simulink model "ConSys_A1"  (Simulink 8.3)
settings: Solver=ode3  StartTime=0.0  StopTime=Time(end)  FixedStep=Ts  RelTol=1e-3
values from neighbouring files (symbols this model uses):
  d = r*h    (= 1.6)    [StartUp_A1.m]
  d0 = d*h    (= 0.0032)    [StartUp_A1.m]
  h = 0.002    [StartUp_A1.m]
  Ka = diag([ 3  20  20  150  355  520])    [StartUp_A1.m]
  Kd = diag([ 3   5  25  100   15 1050])    [StartUp_A1.m]
  Ki = diag([35 555 810 7410 1850 5815])    [StartUp_A1.m]
  Kp = diag([55 180 350 1960  680 4450])    [StartUp_A1.m]
  r = 800    [StartUp_A1.m]
  TD = ss(Atd,Btd,Ctd,Dtd,Ts)    [StartUp_A1.m]
  Ts = 1/200    (= 0.005)    [StartUp_A1.m]
undefined symbols (not defined in the file or in its folder): DiscIntNeverNeededParam
undefined symbols (not defined in the file): ADAMS_cwd, ADAMS_exec, ADAMS_host, ADAMS_init, ADAMS_inputs, ADAMS_outputs, ADAMS_prefix, ADAMS_static, ADAMS_sysdir
libraries: cstblocks x6
(part 1 of 9)
settings Model: Creator=baqumau  LastModifiedBy=baqumau
settings SolverCC: SolverResetMethod=Robust  AutoInsertRateTranBlk=on
settings DataIOCC: SignalLoggingSaveFormat=Dataset
settings DebuggingCC: UnderspecifiedInitializationDetection=Simplified  StateNameClashWarn=none
settings GRTTargetCC: CombineOutputUpdateFcns=on  GRTInterface=off

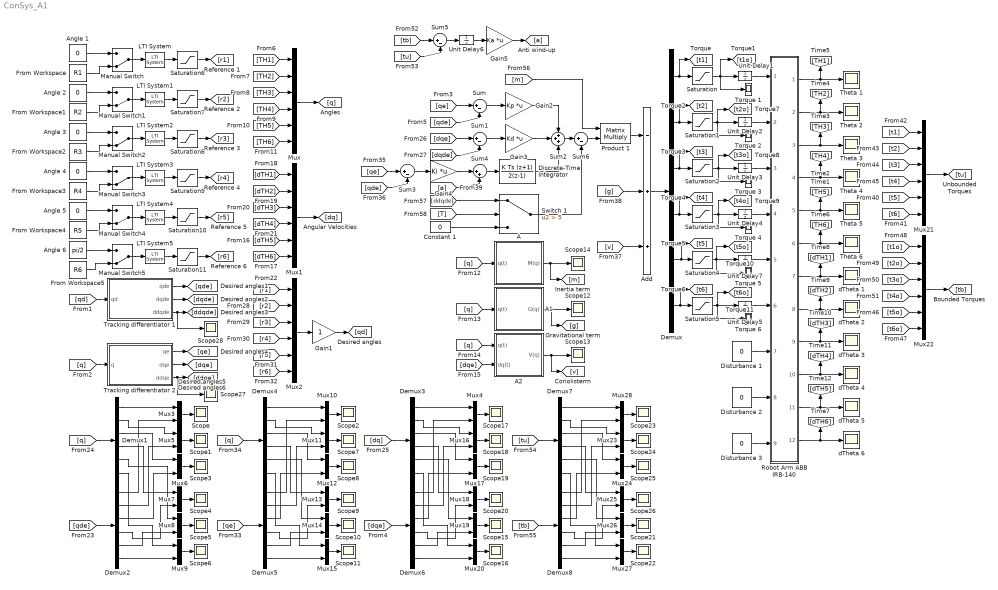
== system ConSys_A1 ==
  A : Subsystem
  A1 : Subsystem
  A2 : Subsystem
  Add : Sum  Inputs=-++
  Angle {1..5} (5 alike) : Constant  Value=0
  Angle 6 : Constant  Value=pi/2
  Constant 1 : Constant  Value=0
  Demux{,1..8} (9 alike) : Demux  Outputs=6
  Discrete-Time Integrator : DiscreteIntegrator  IntegratorMethod=Integration: Trapezoidal  InitialCondition=[0 0 0 0 0 0]'  SampleTime=Ts  ICPrevOutput=DiscIntNeverNeededParam  ICPrevScaledInput=DiscIntNeverNeededParam
  Disturbance 1 : Constant  Value=0
  Disturbance 2 : Constant  Value=0
  Disturbance 3 : Constant  Value=0
  From Workspace : FromWorkspace  VariableName=R1
  From Workspace1 : FromWorkspace  VariableName=R2
  From Workspace2 : FromWorkspace  VariableName=R3
  From Workspace3 : FromWorkspace  VariableName=R4
  From Workspace4 : FromWorkspace  VariableName=R5
  From Workspace5 : FromWorkspace  VariableName=R6
  Gain1 : Gain
  Gain2 : Gain  Gain=Kp  Multiplication=Matrix(K*u)
  Gain3 : Gain  Gain=Kd  Multiplication=Matrix(K*u)
  Gain4 : Gain  Gain=Ki  Multiplication=Matrix(K*u)
  Gain5 : Gain  Gain=Ka  Multiplication=Matrix(K*u)
  LTI System : cstblocks/LTI System  sys=F1z  IC=[]
  LTI System1 : cstblocks/LTI System  sys=F2z  IC=[]
  LTI System2 : cstblocks/LTI System  sys=F3z  IC=[]
  LTI System3 : cstblocks/LTI System  sys=F4z  IC=[]
  LTI System4 : cstblocks/LTI System  sys=F5z  IC=[]
  LTI System5 : cstblocks/LTI System  sys=F6z  IC=[]
  Manual Switch{,1..5} (6 alike) : ManualSwitch  CurrentSetting=0
  Mux{,1..2,21..22} (5 alike) : Mux  Inputs=6
  Mux{3..20,23..28} (24 alike) : Mux  Inputs=2
  Product 1 : Product  Multiplication=Matrix(*)
  Robot Arm ABB IRB-140 : Subsystem
  Saturation : Saturate  UpperLimit=400  LowerLimit=-400
  Saturation1 : Saturate  UpperLimit=300  LowerLimit=-300
  Saturation10 : Saturate  UpperLimit=120  LowerLimit=-120
  Saturation11 : Saturate  UpperLimit=400  LowerLimit=-400
  Saturation2 : Saturate  UpperLimit=250  LowerLimit=-250
  Saturation3 : Saturate  UpperLimit=50  LowerLimit=-50
  Saturation4 : Saturate  UpperLimit=8  LowerLimit=-8
  Saturation5 : Saturate  UpperLimit=0.3  LowerLimit=-0.3
  Saturation6 : Saturate  UpperLimit=180  LowerLimit=-180
  Saturation7 : Saturate  UpperLimit=100  LowerLimit=-100
  Saturation8 : Saturate  UpperLimit=140  LowerLimit=-140
  Saturation9 : Saturate  UpperLimit=200*pi/180  LowerLimit=-200*pi/180
  Scope{,1..28} (29 alike) : Scope
      Scope settings: YMin=-2  YMax=2  SaveName=ScopeData18
      Scope1 settings: YMin=-3  YMax=3  SaveName=ScopeData19
      Scope10 settings: YMin=-2  YMax=2  SaveName=ScopeData20
      Scope11 settings: YMin=-2  SaveName=ScopeData25
      Scope12 settings: YMin=-2  YMax=4  SaveName=ScopeData30
      Scope13 settings: YMin=-2  YMax=4  SaveName=ScopeData31
      Scope14 settings: YMin=-2  YMax=4  SaveName=ScopeData32
      Scope15 settings: YMin=-2  YMax=2  SaveName=ScopeData33
      Scope16 settings: YMin=-2  SaveName=ScopeData34
      Scope17 settings: YMin=-1  YMax=2  SaveName=ScopeData35
      Scope18 settings: YMin=-1  YMax=2  SaveName=ScopeData36
      Scope19 settings: YMin=-1  YMax=2  SaveName=ScopeData37
      Scope2 settings: YMin=-1  YMax=2  SaveName=ScopeData26
      Scope20 settings: YMin=-1  YMax=2  SaveName=ScopeData38
      Scope21 settings: YMin=-2  YMax=2  SaveName=ScopeData39
      Scope22 settings: YMin=-1  YMax=1  SaveName=ScopeData40
      Scope23 settings: YMin=-1  YMax=2  SaveName=ScopeData41
      Scope24 settings: YMin=-1  YMax=2  SaveName=ScopeData42
      Scope25 settings: YMin=-1  YMax=2  SaveName=ScopeData43
      Scope26 settings: YMin=-1  YMax=2  SaveName=ScopeData44
      Scope27 settings: YMin=-2  YMax=2  SaveName=ScopeData45
      Scope28 settings: YMin=-20  YMax=20  SaveName=ScopeData46
      Scope3 settings: YMin=-2  YMax=2  SaveName=ScopeData21
      Scope4 settings: YMin=-2  YMax=2  SaveName=ScopeData22
      Scope5 settings: YMin=-2  YMax=2  SaveName=ScopeData23
      Scope6 settings: SaveName=ScopeData24
      Scope7 settings: YMin=-1  YMax=2  SaveName=ScopeData27
      Scope8 settings: YMin=-1  YMax=2  SaveName=ScopeData28
      Scope9 settings: YMin=-1  YMax=2  SaveName=ScopeData29
  Sum{,1,3,5..6} (5 alike) : Sum  Inputs=|+-
  Sum2 : Sum  Inputs=+++
  Sum4 : Sum  Inputs=|++
  Switch 1 : Switch  Criteria=u2 > Threshold  Threshold=5
  Theta {1..6} (6 alike) : Scope
      Theta 1 settings: YMin=-0.6  YMax=0.6
      Theta 2 settings: YMin=-1  YMax=1  SaveName=ScopeData2
      Theta 3 settings: SaveName=ScopeData3
      Theta 4 settings: SaveName=ScopeData4
      Theta 5 settings: SaveName=ScopeData5
      Theta 6 settings: YMin=-100  YMax=100
  Torque {1..6} (6 alike) : Scope
      Torque 1 settings: YMin=-400  YMax=400  SaveName=ScopeData6
      Torque 2 settings: YMin=-400  YMax=400  SaveName=ScopeData7
      Torque 3 settings: YMin=-400  YMax=400  SaveName=ScopeData8
      Torque 4 settings: YMin=-20  YMax=20  SaveName=ScopeData9
      Torque 5 settings: YMin=-400  YMax=400  SaveName=ScopeData10
      Torque 6 settings: YMin=-0.3  YMax=0.3  SaveName=ScopeData11
  Tracking differentiator 1 : Subsystem
  Tracking differentiator 2 : Subsystem
  Unit Delay{1..7} (7 alike) : UnitDelay  SampleTime=-1
  dTheta {1..6} (6 alike) : Scope
      dTheta 1 settings: SaveName=ScopeData13
      dTheta 2 settings: SaveName=ScopeData14
      dTheta 3 settings: SaveName=ScopeData15
      dTheta 4 settings: SaveName=ScopeData16
      dTheta 5 settings: SaveName=ScopeData17
      dTheta 6 settings: SaveName=ScopeData12
  wires:
  Disturbance 2/1 -> Robot Arm ABB IRB-140/8(Disturbance_2)
  Saturation1/1 -> Torque 2/1, Unit Delay2/1, [t2o]
  Saturation2/1 -> Torque 3/1, Unit Delay3/1, [t3o]
  Saturation3/1 -> Unit Delay4/1, Torque 4/1, [t4o]
  Saturation4/1 -> Unit Delay7/1, [t5o], Torque 5/1
  Saturation5/1 -> Unit Delay5/1, Torque 6/1, [t6o]
  [TH3] -> Mux/3
  [TH6] -> Mux/6
  [TH1] -> Mux/1
  [TH4] -> Mux/4
  [TH5] -> Mux/5
  [TH2] -> Mux/2
  Mux/1 -> [q]
  [q] -> A/1(q(t))
  [q] -> A1/1(q(t))
  [dTH3] -> Mux1/3
  [dTH6] -> Mux1/6
  [dTH1] -> Mux1/1
  [dTH4] -> Mux1/4
  [dTH5] -> Mux1/5
  [dTH2] -> Mux1/2
  Mux1/1 -> [dq]
  Mux2/1 -> Gain1/1
  Demux/1 -> Saturation/1, [t1]
  Demux/2 -> Saturation1/1, [t2]
  Demux/3 -> Saturation2/1, [t3]
  Demux/4 -> Saturation3/1, [t4]
  Demux/6 -> [t6], Saturation5/1
  [qd] -> Tracking differentiator 1/1(qd)
  Tracking differentiator 1/1(qde) -> [qde]
  Tracking differentiator 1/2(dqde) -> [dqde]
  Tracking differentiator 1/3(ddqde) -> Scope28/1, [ddqde]
  [q] -> Demux1/1
  [qde] -> Demux2/1
  Mux3/1 -> Scope/1
  Saturation/1 -> Unit Delay1/1, Torque 1/1, [t1o]
  [q] -> A2/1(q(t))
  [dqe] -> A2/2(dq(t))
  Mux5/1 -> Scope1/1
  Mux6/1 -> Scope3/1
  Mux7/1 -> Scope4/1
  Mux8/1 -> Scope5/1
  Mux9/1 -> Scope6/1
  Demux1/1 -> Mux3/1
  Demux2/1 -> Mux3/2
  Demux1/2 -> Mux5/1
  Demux2/2 -> Mux5/2
  Demux1/3 -> Mux6/1
  Demux2/3 -> Mux6/2
  Demux1/4 -> Mux7/1
  Demux2/4 -> Mux7/2
  Demux1/5 -> Mux8/1
  Demux2/5 -> Mux8/2
  Demux1/6 -> Mux9/1
  Demux2/6 -> Mux9/2
  [r1] -> Mux2/1
  [qe] -> Sum/1
  [qde] -> Sum/2
  Angle 1/1 -> Manual Switch/1
  From Workspace/1 -> Manual Switch/2
  Manual Switch/1 -> LTI System/1
  Angle 2/1 -> Manual Switch1/1
  From Workspace1/1 -> Manual Switch1/2
  Manual Switch1/1 -> LTI System1/1
  Angle 3/1 -> Manual Switch2/1
  From Workspace2/1 -> Manual Switch2/2
  Manual Switch2/1 -> LTI System2/1
  Angle 4/1 -> Manual Switch3/1
  From Workspace3/1 -> Manual Switch3/2
  Manual Switch3/1 -> LTI System3/1
  Angle 5/1 -> Manual Switch4/1
  From Workspace4/1 -> Manual Switch4/2
  Manual Switch4/1 -> LTI System4/1
  Angle 6/1 -> Manual Switch5/1
  From Workspace5/1 -> Manual Switch5/2
  Manual Switch5/1 -> LTI System5/1
  [q] -> Demux4/1
  [qe] -> Demux5/1
  Mux10/1 -> Scope2/1
  Mux11/1 -> Scope7/1
  Mux12/1 -> Scope8/1
  Mux13/1 -> Scope9/1
  Mux14/1 -> Scope10/1
  Mux15/1 -> Scope11/1
  Demux4/1 -> Mux10/1
  Demux5/1 -> Mux10/2
  Demux4/2 -> Mux11/1
  Demux5/2 -> Mux11/2
  Demux4/3 -> Mux12/1
  Demux5/3 -> Mux12/2
  Demux4/4 -> Mux13/1
  Demux5/4 -> Mux13/2
  Demux4/5 -> Mux14/1
  Demux5/5 -> Mux14/2
  Demux4/6 -> Mux15/1
  Demux5/6 -> Mux15/2
  Saturation6/1 -> [r1]
  LTI System/1 -> Saturation6/1
  LTI System1/1 -> Saturation7/1
  LTI System2/1 -> Saturation8/1
  LTI System3/1 -> Saturation9/1
  LTI System4/1 -> Saturation10/1
  LTI System5/1 -> Saturation11/1
  Saturation7/1 -> [r2]
  Saturation8/1 -> [r3]
  Saturation9/1 -> [r4]
  Saturation10/1 -> [r5]
  Saturation11/1 -> [r6]
  Disturbance 1/1 -> Robot Arm ABB IRB-140/7(Disturbance_1)
  Disturbance 3/1 -> Robot Arm ABB IRB-140/9(Disturbance_3)
  [q] -> Tracking differentiator 2/1(q)
  Tracking differentiator 2/1(qe) -> [qe]
  Tracking differentiator 2/2(dqe) -> [dqe]
  Tracking differentiator 2/3(ddqe) -> Scope27/1, [ddqe]
  A1/1(G(q)) -> [g], Scope12/1
  A2/1(V(q)) -> [v], Scope13/1
  A/1(M(q)) -> [m], Scope14/1
  Gain1/1 -> [qd]
  [r2] -> Mux2/2
  [r3] -> Mux2/3
  [r4] -> Mux2/4
  [r5] -> Mux2/5
  [r6] -> Mux2/6
  [dq] -> Demux3/1
  [dqe] -> Demux6/1
  Mux4/1 -> Scope17/1
  Mux16/1 -> Scope18/1
  Mux17/1 -> Scope19/1
  Mux18/1 -> Scope20/1
  Mux19/1 -> Scope15/1
  Mux20/1 -> Scope16/1
  Demux3/1 -> Mux4/1
  Demux6/1 -> Mux4/2
  Demux3/2 -> Mux16/1
  Demux6/2 -> Mux16/2
  Demux3/3 -> Mux17/1
  Demux6/3 -> Mux17/2
  Demux3/4 -> Mux18/1
  Demux6/4 -> Mux18/2
  Demux3/5 -> Mux19/1
  Demux6/5 -> Mux19/2
  Demux3/6 -> Mux20/1
  Demux6/6 -> Mux20/2
  Sum/1 -> Gain2/1
  [dqe] -> Sum1/1
  [dqde] -> Sum1/2
  Sum1/1 -> Gain3/1
  [qe] -> Sum3/1
  [qde] -> Sum3/2
  Unit Delay1/1 -> Robot Arm ABB IRB-140/1(Torque_1)
  Unit Delay2/1 -> Robot Arm ABB IRB-140/2(Torque_2)
  Demux/5 -> [t5], Saturation4/1
  Sum3/1 -> Gain4/1
  Gain4/1 -> Sum4/1
  Sum4/1 -> Discrete-Time Integrator/1
  [a] -> Sum4/2
  [t3] -> Mux21/3
  [t1] -> Mux21/1
  [t4] -> Mux21/4
  [t5] -> Mux21/5
  [t2] -> Mux21/2
  Mux21/1 -> [tu]
  [t6] -> Mux21/6
  [t3o] -> Mux22/3
  [t1o] -> Mux22/1
  [t4o] -> Mux22/4
  [t5o] -> Mux22/5
  [t2o] -> Mux22/2
  Mux22/1 -> [tb]
  [t6o] -> Mux22/6
  [tb] -> Sum5/1
  [tu] -> Sum5/2
  Gain5/1 -> [a]
  Unit Delay6/1 -> Gain5/1
  Sum5/1 -> Unit Delay6/1
  [tu] -> Demux7/1
  [tb] -> Demux8/1
  Mux28/1 -> Scope23/1
  Mux23/1 -> Scope24/1
  Mux24/1 -> Scope25/1
  Mux25/1 -> Scope26/1
  Mux26/1 -> Scope21/1
  Mux27/1 -> Scope22/1
  Demux7/1 -> Mux28/1
  Demux8/1 -> Mux28/2
  Demux7/2 -> Mux23/1
  Demux8/2 -> Mux23/2
  Demux7/3 -> Mux24/1
  Demux8/3 -> Mux24/2
  Demux7/4 -> Mux25/1
  Demux8/4 -> Mux25/2
  Demux7/5 -> Mux26/1
  Demux8/5 -> Mux26/2
  Demux7/6 -> Mux27/1
  Demux8/6 -> Mux27/2
  Add/1 -> Demux/1
  Gain2/1 -> Sum2/1
  Gain3/1 -> Sum2/2
  Discrete-Time Integrator/1 -> Sum2/3
  [m] -> Product 1/1
  [ddqde] -> Switch 1/1
  Sum2/1 -> Sum6/1
  Sum6/1 -> Product 1/2
  Product 1/1 -> Add/1
  [g] -> Add/2
  [v] -> Add/3
  Unit Delay3/1 -> Robot Arm ABB IRB-140/3(Torque_3)
  [T] -> Switch 1/2
  Constant 1/1 -> Switch 1/3
  Switch 1/1 -> Sum6/2
  Unit Delay4/1 -> Robot Arm ABB IRB-140/4(Torque_4)
  Unit Delay7/1 -> Robot Arm ABB IRB-140/5(Torque_5)
  Unit Delay5/1 -> Robot Arm ABB IRB-140/6(Torque_6)
  Robot Arm ABB IRB-140/12(dTheta_6) -> [dTH6], dTheta 6/1
  Robot Arm ABB IRB-140/11(dTheta_5) -> [dTH5], dTheta 5/1
  Robot Arm ABB IRB-140/10(dTheta_4) -> [dTH4], dTheta 4/1
  Robot Arm ABB IRB-140/9(dTheta_3) -> [dTH3], dTheta 3/1
  Robot Arm ABB IRB-140/8(dTheta_2) -> [dTH2], dTheta 2/1
  Robot Arm ABB IRB-140/7(dTheta_1) -> [dTH1], dTheta 1/1
  Robot Arm ABB IRB-140/1(Theta_1) -> [TH1], Theta 1/1
  Robot Arm ABB IRB-140/2(Theta_2) -> [TH2], Theta 2/1
  Robot Arm ABB IRB-140/3(Theta_3) -> [TH3], Theta 3/1
  Robot Arm ABB IRB-140/4(Theta_4) -> [TH4], Theta 4/1
  Robot Arm ABB IRB-140/6(Theta_6) -> [TH6], Theta 6/1
  Robot Arm ABB IRB-140/5(Theta_5) -> [TH5], Theta 5/1

== system ConSys_A1/A ==
  q(t) : Inport
  Display : Display
  MATLAB Function 1 : MATLAB Function  TreatAsAtomicUnit=on
  MATLAB Function 2 : MATLAB Function  TreatAsAtomicUnit=on
  MATLAB Function 3 : MATLAB Function  TreatAsAtomicUnit=on
  MATLAB Function 4 : MATLAB Function  TreatAsAtomicUnit=on
  MATLAB Function 5 : MATLAB Function  TreatAsAtomicUnit=on
  MATLAB Function 6 : MATLAB Function  TreatAsAtomicUnit=on
  Math Function : Math  Operator=transpose  SaturateOnIntegerOverflow=on
  Matrix Concatenate : Concatenate  NumInputs=6  Mode=Multidimensional array  ConcatenateDimension=2
  Vector Concatenate{1..6} (6 alike) : Concatenate  NumInputs=6
  M(q) : Outport
  wires:
  Matrix Concatenate/1 -> Math Function/1
  q(t)/1 -> MATLAB Function 3/1(q), MATLAB Function 6/1(q), MATLAB Function 5/1(q), MATLAB Function 4/1(q), MATLAB Function 2/1(q), MATLAB Function 1/1(q)
  Math Function/1 -> Display/1, M(q)/1
  MATLAB Function 1/1(M11) -> Vector Concatenate4/1
  MATLAB Function 1/2(M12) -> Vector Concatenate1/1, Vector Concatenate4/2
  MATLAB Function 1/3(M13) -> Vector Concatenate2/1, Vector Concatenate4/3
  MATLAB Function 1/4(M14) -> Vector Concatenate3/1, Vector Concatenate4/4
  Vector Concatenate4/1 -> Matrix Concatenate/1
  MATLAB Function 2/1(M22) -> Vector Concatenate1/2
  MATLAB Function 2/2(M23) -> Vector Concatenate2/2, Vector Concatenate1/3
  MATLAB Function 2/3(M24) -> Vector Concatenate3/2, Vector Concatenate1/4
  MATLAB Function 2/4(M25) -> Vector Concatenate5/2, Vector Concatenate1/5
  Vector Concatenate1/1 -> Matrix Concatenate/2
  MATLAB Function 3/4(M36) -> Vector Concatenate6/3, Vector Concatenate2/6
  MATLAB Function 3/3(M35) -> Vector Concatenate5/3, Vector Concatenate2/5
  MATLAB Function 3/1(M33) -> Vector Concatenate2/3
  MATLAB Function 3/2(M34) -> Vector Concatenate3/3, Vector Concatenate2/4
  Vector Concatenate2/1 -> Matrix Concatenate/3
  MATLAB Function 4/1(M44) -> Vector Concatenate3/4
  MATLAB Function 4/3(M46) -> Vector Concatenate6/4, Vector Concatenate3/6
  MATLAB Function 4/2(M45) -> Vector Concatenate5/4, Vector Concatenate3/5
  Vector Concatenate3/1 -> Matrix Concatenate/4
  MATLAB Function 1/5(M15) -> Vector Concatenate5/1, Vector Concatenate4/5
  MATLAB Function 5/2(M56) -> Vector Concatenate6/5, Vector Concatenate5/6
  MATLAB Function 5/1(M55) -> Vector Concatenate5/5
  Vector Concatenate5/1 -> Matrix Concatenate/5
  MATLAB Function 6/1(M66) -> Vector Concatenate6/6
  MATLAB Function 1/6(M16) -> Vector Concatenate6/1, Vector Concatenate4/6
  MATLAB Function 2/5(M26) -> Vector Concatenate6/2, Vector Concatenate1/6
  Vector Concatenate6/1 -> Matrix Concatenate/6

== system ConSys_A1/A1 ==
  q(t) : Inport
  Display : Display
  MATLAB Function 1 : MATLAB Function  TreatAsAtomicUnit=on
  Vector Concatenate4 : Concatenate  NumInputs=6
  G(q) : Outport
  wires:
  MATLAB Function 1/6(G61) -> Vector Concatenate4/6
  MATLAB Function 1/5(G51) -> Vector Concatenate4/5
  MATLAB Function 1/4(G41) -> Vector Concatenate4/4
  MATLAB Function 1/3(G31) -> Vector Concatenate4/3
  MATLAB Function 1/2(G21) -> Vector Concatenate4/2
  MATLAB Function 1/1(G11) -> Vector Concatenate4/1
  Vector Concatenate4/1 -> G(q)/1, Display/1
  q(t)/1 -> MATLAB Function 1/1(q)

== system ConSys_A1/A2 ==
  q(t) : Inport
  dq(t) : Inport  Port=2
  Display : Display
  MATLAB Function 1 : MATLAB Function  TreatAsAtomicUnit=on
  MATLAB Function 2 : MATLAB Function  TreatAsAtomicUnit=on
  MATLAB Function 3 : MATLAB Function  TreatAsAtomicUnit=on
  MATLAB Function 4 : MATLAB Function  TreatAsAtomicUnit=on
  MATLAB Function 5 : MATLAB Function  TreatAsAtomicUnit=on
  MATLAB Function 6 : MATLAB Function  TreatAsAtomicUnit=on
  Vector Concatenate4 : Concatenate  NumInputs=6
  V(q) : Outport
  wires:
  q(t)/1 -> MATLAB Function 1/1(q), MATLAB Function 6/1(q), MATLAB Function 5/1(q), MATLAB Function 4/1(q), MATLAB Function 3/1(q), MATLAB Function 2/1(q)
  Vector Concatenate4/1 -> Display/1, V(q)/1
  dq(t)/1 -> MATLAB Function 6/2(dq), MATLAB Function 5/2(dq), MATLAB Function 4/2(dq), MATLAB Function 3/2(dq), MATLAB Function 2/2(dq), MATLAB Function 1/2(dq)
  MATLAB Function 1/1(V1) -> Vector Concatenate4/1
  MATLAB Function 2/1(V2) -> Vector Concatenate4/2
  MATLAB Function 3/1(V3) -> Vector Concatenate4/3
  MATLAB Function 4/1(V4) -> Vector Concatenate4/4
  MATLAB Function 5/1(V5) -> Vector Concatenate4/5
  MATLAB Function 6/1(V6) -> Vector Concatenate4/6

== system ConSys_A1/Robot Arm ABB IRB-140 ==
  Torque_1 : Inport
  Torque_2 : Inport  Port=2
  Torque_3 : Inport  Port=3
  Torque_4 : Inport  Port=4
  Torque_5 : Inport  Port=5
  Torque_6 : Inport  Port=6
  Disturbance_1 : Inport  Port=7
  Disturbance_2 : Inport  Port=8
  Disturbance_3 : Inport  Port=9
  ADAMS Plant : Subsystem  LoadFcn=|  InitFcn=clear mex  mask(Adams Plant){exevie=ADAMS_sysdir, nam_in=ADAMS_inputs, namout=ADAMS_outputs, nampre=ADAMS_prefix, outfil=ADAMS_prefix, exesol=ADAMS_exec, stat=ADAMS_static, inicmd=[ADAMS_init], exetyp=C++, comtyp=PIPE(DDE), workdir=ADAMS_cwd, ada_host=ADAMS_host, modani=batch, modsim=discrete, dft=no, simulink_lead_cosim=yes, pin_interp_order=0, pout_extrap_order=0, pin_extrap_order=0, pout_interp_order=0, dt_out=Ts, o_rate=1, more=off}
      | %check based on dialog box setting for when setting by popup menu                                             
      | if exist('ADAMS_solver_type')                                                                                 
      |   if strcmp(ADAMS_solver_type,'C++')                                                                          
      |     set_param(gcb,'exetyp','C++');                                                                            
      |   else                                                                                                        
      |     set_param(gcb,'exetyp','Fortran');                                                                        
      |   end                                                                                                         
      | else                                                                                                          
      |   set_param(gcb,'exetyp','C++');                                                                              
      | end                                                                                                           
      | %set the mode if using acar_solver                                                                            
      | %REQUIRED HERE BECAUSE BELOW CAUSES MDLTERMINATE TO BE CALLED 2 TIMES IN MIDDLE OF SIMULATION WHEN SET IN MASK
      |                                                                                                               
      | %enable the direct feedthrough, sim mode, anim mode parameters by default                                     
      |                                                                                                               
      | if exist('set_some_params_states')                                                                            
      |                                                                                                               
      |   set_some_params_states({'dft','modsim','modani'},{'on','on','on'},'MaskEnables',gcb)                        
      |   %turn on direct feedthrough option                                                                          
      |   set_some_params_states({'dft'},{'on'},'MaskVisibilities',gcb)                                               
      |                                                                                                               
      |  end                                                                                                          
      |                                                                                                               
      |                                                                                                               
      | if exist('ADAMS_exec')                                                                                        
      |   if and(strcmp(get_param(gcb,'exesol'),'ADAMS_exec'),strcmp(ADAMS_exec,'acar_solver'))                       
      |     %set the sim mode to discrete -- only supported mode                                                      
      |     set_param(gcb,'modsim','discrete')                                                                        
      |      %turn off direct feedthrough option                                                                      
      |      set_some_params_states({'dft'},{'off'},'MaskVisibilities',gcb)                                           
      |     %set the animation mode to batch -- only supported mode                                                   
      |     set_param(gcb,'modani','batch')                                                                           
      |     %disable the direct feedthrough, sim mode, anim mode parameters                                           
      |     set_some_params_states({'modsim','modani'},{'off','off'},'MaskEnables',gcb)                               
      |   end
      |   if and(strcmp(get_param(gcb,'exesol'),'ADAMS_exec'),strcmp(ADAMS_exec,'apre_solver'))                       
      |     %set the sim mode to discrete -- only supported mode                                                      
      |     set_param(gcb,'modsim','discrete')                                                                        
      |      %turn off direct feedthrough option                                                                      
      |      set_some_params_states({'dft'},{'off'},'MaskVisibilities',gcb)                                           
      |     %set the animation mode to batch -- only supported mode                                                   
      |     set_param(gcb,'modani','batch')                                                                           
      |     %disable the direct feedthrough, sim mode, anim mode parameters                                           
      |     set_some_params_states({'modsim','modani'},{'off','off'},'MaskEnables',gcb)                               
      |   end                                                                                                  
      | end
      mask prompts: exevie "Adams install directory"; nam_in "Adams View input names"; namout "Adams View output names"; nampre "Adams model file prefix"; outfil "Output files prefix (opt.: if blank - no output)"; exesol "User executable (opt.: if blank - use standard)"; stat "Initial static simulation flag"; inicmd "Initialization commands"; exetyp "Adams Solver type"; comtyp "Interprocess option"; workdir "Adams working directory"; ada_host "Adams host"; modani "Animation mode"; modsim "Simulation mode"; dft "Direct feedthrough"; simulink_lead_cosim "Discrete Computational Order - Simulink Leads Adams"; pin_interp_order "Plant input interpolation order"; pout_extrap_order "Plant output extrapolation order"; pin_extrap_order "Plant input extrapolation order"; pout_interp_order "Plant output interpolation order"; dt_out "Communication interval"; o_rate "Number of communications per output step"; more "More parameters"
      mask help: Simulate any Adams plant model either in Adams Solver form (.adm file) or in Adams View form (.cmd file)
      settings: OpenFcn=|
      | open_system(gcb,'mask')
      | if not(exist('set_some_params_states'))
      | 
      | warning('The script "set_some_params_states.m" cannot be found in the MATLAB PATH.  Cannot update the ADAMS Plant S-Function parameters.')
      | 
      | warning('Recommended action(optional):  run the Adams Controls .m file first to help choose the correct settings in the Adams S-Function block.')
      | 
      | end
      mask Help:
      | <html>
      | This S-Function represents the non-linear Adams Plant with the inputs sent to the Adams model <br>
      |  and the outputs generated by the Adams model.  See the Adams Controls documentation for more <br>
      | information.  This plant uses the following variables:<br>
      | <br>
      | <b>ADAMS_sysdir  :</b> Adams installation directory<br>
      | <b>ADAMS_inputs  :</b> Input variables View names vector<br>
      | <b>ADAMS_outputs :</b> Outputs variables View names vector<br>
      | <b>ADAMS_prefix  : </b>ADAMS model files prefix (.adm, .cmd); also doubles as output files prefix<br>
      | <b>ADAMS_exec :</b> Adams Solver user library or keyword (e.g., acar_solver)<br>
      | <b>ADAMS_static :</b> yes|no - initial static before Co-simulation(discrete)/Function Evaluation(continuous)<br>
      | <b>ADAMS_init :</b>Initialization commands (i.e., Adams View or Solver commands, depending on setting for Animation mode)<br>
      | <b>ADAMS_cwd : </b> Current working directory (for TCP/IP)<br>
      | <b>ADAMS_host : </b>Name of Adams server host (for TCP/IP)<br>
      | <b>ADAMS_mode :</b> Linear or non-linear (i.e., co-sim, function eval)<br>
      | <b>ADAMS_solver_type :</b>Fortran or C++ (used to set popup menu when first loaded) <br>
      | 
      | 
      | <br>
      | The following settings can be chosen:<br>
      | <br>
      | <b>Adams Solver type:</b>  Fortran or C++ (will also set ADAMS_solver_type)<br>
      | <b>Interprocess option:</b> Pipe(DDE), TCP/IP or DIRECT; TCP/IP can allow different machines run Adams and MATLAB<br>
      | <b>Animation mode:</b> batch (Solver, uses .adm) or interactive (View, uses .cmd)<br>
      | <b>Simulation mode:</b> discrete (Co-simulation) or continuous (Function Evaluation)<br>
      | <b>Discrete Computational Order - Simulink Lead Adams:</b> for discrete mode, chooses if Simulink leads the integration (yes) or lags (no);<br> if set to "no", can remove algebraic loop<br>
      | <b>Plant input interpolation order:</b> 0 = zero-order hold; 1 = linear (discrete mode only, where Simulink leads)<br>
      | <b>Plant output extrapolation order:</b> 0 = zero-order hold;1 = linear(discrete mode only, where Simulink leads)<br>
      | <b>Plant input extrapolation order:</b> 0 = zero-order hold; 1 = linear (discrete mode only, where Adams leads)<br>
      | <b>Plant output interpolation order:</b> 0 = zero-order hold;1 = linear(discrete mode only, where Adams leads)<br>
      | <b>Direct feedthrough:</b> yes|no - yes = Input directly effect output(continuous mode-only)<br>
      | <b>Communication interval:</b> Time step at which Co-simulation exchange information (e.g.,0.005); also controls <br>output for continuous mode (Function Evaluation)<br>
      | <b>Number of communications per output step: </b>Sets Adams output rate (.res, .req, .gra) integer value (default: 1)<br>
      | </html>
      mask Callback exesol:
      | if exist('set_some_params_states')
      | %enable the direct feedthrough, sim mode, anim mode parameters
      | set_some_params_states({'dft','modsim','modani'},{'on','on','on'},'MaskEnables',gcb)
      | %turn on direct feedthrough option
      | set_some_params_states({'dft'},{'on'},'MaskVisibilities',gcb)
      | end
      | 
      | if exist('ADAMS_exec')
      |   if and(strcmp(get_param(gcb,'exesol'),'ADAMS_exec'),strcmp(ADAMS_exec,'acar_solver'))
      |     %set the sim mode to discrete -- only supported mode
      |     %REMOVED:  BELOW CAUSES MDLTERMINATE TO BE CALLED 2 TIMES IN MIDDLE OF SIMULATION
      |     %Now in LoadFcn callback
      |     %set_param(gcb,'modsim','discrete')
      |      %turn off direct feedthrough option
      |     set_some_params_states({'dft'},{'off'},'MaskVisibilities',gcb)
      |     %set the animation mode to batch -- only supported mode
      |     %REMOVED:  BELOW CAUSES MDLTERMINATE TO BE CALLED 2 TIMES IN MIDDLE OF SIMULATION
      |     %Now in LoadFcn callback
      |     %set_param(gcb,'modani','batch')
      |     %disable the direct feedthrough, sim mode, anim mode parameters
      |     set_some_params_states({'modsim','modani'},{'off','off'},'MaskEnables',gcb)
      |   end
      | end
      mask TypeOptions exetyp: Fortran | C++
      mask Callback exetyp:
      | if strcmp(get_param(gcb,'exetyp'),'C++')
      |     ADAMS_solver_type='C++';
      | else
      |     ADAMS_solver_type='Fortran';
      | end
      mask TypeOptions comtyp: PIPE(DDE) | TCP/IP | DIRECT
      mask Callback comtyp:
      | if exist('set_some_params_states')
      | if strcmp(get_param(gcb,'comtyp'),'PIPE(DDE)') || strcmp(get_param(gcb,'comtyp'),'DIRECT')
      |     %turn off cwd, host options
      |     set_some_params_states({'ada_host','workdir'},{'off','off'},'MaskVisibilities',gcb)
      | else%if strcmp(get_param(gcb,'modsim'),'TCP/IP')
      |     %turn on cwd, host options
      |     set_some_params_states({'ada_host','workdir'},{'on','on'},'MaskVisibilities',gcb)
      | end
      | end
      mask TypeOptions modani: batch | interactive
      mask TypeOptions modsim: discrete | continuous
      mask Callback modsim:
      | if exist('set_some_params_states')
      | if strcmp(get_param(gcb,'modsim'),'discrete')
      |      %turn off direct feedthrough option
      |     set_some_params_states({'dft'},{'off'},'MaskVisibilities',gcb)
      |     %turn on discrete co-sim type if want to see more
      |     if strcmp(get_param(gcb,'more'),'on')
      |         set_some_params_states({'simulink_lead_cosim'},{'on'},'MaskVisibilities',gcb)
      |     end
      |     if strcmp(get_param(gcb,'simulink_lead_cosim'),'yes')
      |         %turn on interpolation/extrapolation options
      |         set_some_params_states({'pin_interp_order','pout_extrap_order',},{'on','on'},'MaskVisibilities',gcb)
      |     else
      |         set_some_params_states({'pin_extrap_order','pout_interp_order'},{'on','on'},'MaskVisibilities',gcb)
      |     end
      | else%if strcmp(get_param(gcb,'modsim'),'continuous')
      |      %turn off direct feedthrough option
      |     set_some_params_states({'dft'},{'on'},'MaskVisibilities',gcb)
      |     %turn off interpolation/extrapolation options
      |     set_some_params_states({'pin_interp_order','pout_extrap_order','pin_extrap_order','pout_interp_order','simulink_lead_cosim'},{'off','off','off','off','off'},'MaskVisibilities',gcb)
      | end
      | end
      mask TypeOptions dft: no | yes
      mask TypeOptions simulink_lead_cosim: yes | no
      mask Callback simulink_lead_cosim:
      | if exist('set_some_params_states')
      | if (strcmp(get_param(gcb,'simulink_lead_cosim'),'yes') && strcmp(get_param(gcb,'modsim'),'discrete'))
      |      %turn off unused interpolate/extrapolate options
      |     set_some_params_states({'pin_extrap_order','pout_interp_order'},{'off','off'},'MaskVisibilities',gcb)
      |     %turn on used interpolate/extrapolate options
      |     set_some_params_states({'pin_interp_order','pout_extrap_order'},{'on','on'},'MaskVisibilities',gcb)
      | elseif (strcmp(get_param(gcb,'simulink_lead_cosim'),'no') && strcmp(get_param(gcb,'modsim'),'discrete'))
      |     %turn on used interpolate/extrapolate options
      |     set_some_params_states({'pin_extrap_order','pout_interp_order'},{'on','on'},'MaskVisibilities',gcb)
      |      %turn off unused interpolate/extrapolate options
      |     set_some_params_states({'pin_interp_order','pout_extrap_order'},{'off','off'},'MaskVisibilities',gcb)
      | end
      | end
      mask TypeOptions pin_interp_order: 0 | 1
      mask TypeOptions pout_extrap_order: 0 | 1
      mask TypeOptions pin_extrap_order: 0 | 1
      mask TypeOptions pout_interp_order: 0 | 1
      mask Callback more:
      | if exist('set_some_params_states')
      | if (strcmp(get_param(gcb,'more'),'on'))
      |      %turn on infrequently used options
      |     set_some_params_states({'exevie','nam_in','namout','exesol','stat','inicmd'},{'on','on','on','on','on','on'},'MaskVisibilities',gcb)
      |     if strcmp(get_param(gcb,'modsim'),'discrete')
      |         set_some_params_states({'simulink_lead_cosim'},{'on'},'MaskVisibilities',gcb)
      |     end
      | elseif (strcmp(get_param(gcb,'more'),'off'))
      |     %turn off infrequently used options
      |     set_some_params_states({'exevie','nam_in','namout','exesol','stat','inicmd'},{'off','off','off','off','off','off'},'MaskVisibilities',gcb)
      |     if strcmp(get_param(gcb,'modsim'),'discrete')
      |         set_some_params_states({'simulink_lead_cosim'},{'off'},'MaskVisibilities',gcb)
      |     end
      | end
      | end
      mask Display: disp( 'MSC Software' )
  Clock : Clock
  Demux : Demux  Outputs=12
  Mux : Mux  Inputs=9
  T To Workspace : ToWorkspace  VariableName=ADAMS_tout
      settings: MaxDataPoints=100000
  U To Workspace : ToWorkspace  VariableName=ADAMS_uout
      settings: MaxDataPoints=100000
  Y To Workspace : ToWorkspace  VariableName=ADAMS_yout
      settings: MaxDataPoints=100000
  Theta_1 : Outport
  Theta_2 : Outport  Port=2
  Theta_3 : Outport  Port=3
  Theta_4 : Outport  Port=4
  Theta_5 : Outport  Port=5
  Theta_6 : Outport  Port=6
  dTheta_1 : Outport  Port=7
  dTheta_2 : Outport  Port=8
  dTheta_3 : Outport  Port=9
  dTheta_4 : Outport  Port=10
  dTheta_5 : Outport  Port=11
  dTheta_6 : Outport  Port=12
  wires:
  Disturbance_3/1 -> Mux/9
  Disturbance_2/1 -> Mux/8
  Disturbance_1/1 -> Mux/7
  Torque_6/1 -> Mux/6
  Torque_5/1 -> Mux/5
  Torque_4/1 -> Mux/4
  Torque_3/1 -> Mux/3
  Torque_2/1 -> Mux/2
  Torque_1/1 -> Mux/1
  Demux/12 -> dTheta_6/1
  Demux/11 -> dTheta_5/1
  Demux/10 -> dTheta_4/1
  Demux/9 -> dTheta_3/1
  Demux/8 -> dTheta_2/1
  Demux/7 -> dTheta_1/1
  Demux/6 -> Theta_6/1
  Demux/5 -> Theta_5/1
  Demux/4 -> Theta_4/1
  Demux/3 -> Theta_3/1
  Demux/2 -> Theta_2/1
  Demux/1 -> Theta_1/1
  ADAMS Plant/1(ADAMS outputs) -> Y To Workspace/1, Demux/1
  Mux/1 -> U To Workspace/1, ADAMS Plant/1(ADAMS inputs)
  Clock/1 -> T To Workspace/1

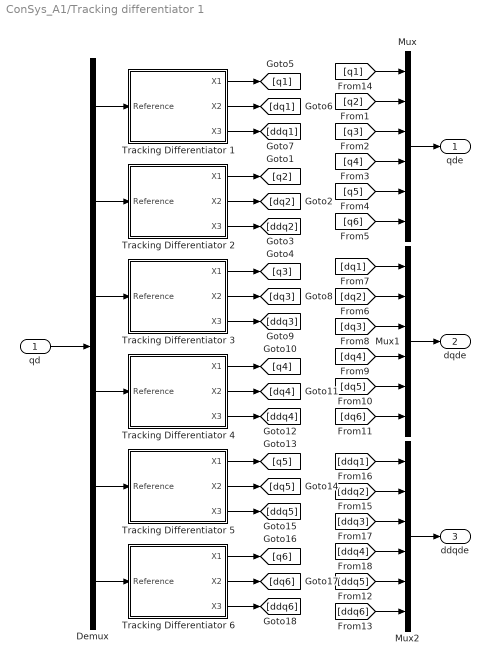
== system ConSys_A1/Tracking differentiator 1 ==
  qd : Inport
  Demux : Demux  Outputs=6
  Mux : Mux  Inputs=6
  Mux1 : Mux  Inputs=6
  Mux2 : Mux  Inputs=6
  Tracking Differentiator 1 : Subsystem
  Tracking Differentiator 2 : Subsystem
  Tracking Differentiator 3 : Subsystem
  Tracking Differentiator 4 : Subsystem
  Tracking Differentiator 5 : Subsystem
  Tracking Differentiator 6 : Subsystem
  qde : Outport
  dqde : Outport  Port=2
  ddqde : Outport  Port=3
  wires:
  Tracking Differentiator 1/1(X1) -> [q1]
  Tracking Differentiator 1/2(X2) -> [dq1]
  Tracking Differentiator 1/3(X3) -> [ddq1]
  Tracking Differentiator 2/1(X1) -> [q2]
  Tracking Differentiator 2/2(X2) -> [dq2]
  Tracking Differentiator 2/3(X3) -> [ddq2]
  qd/1 -> Demux/1
  Demux/1 -> Tracking Differentiator 1/1(Reference)
  Demux/2 -> Tracking Differentiator 2/1(Reference)
  Tracking Differentiator 3/1(X1) -> [q3]
  Tracking Differentiator 3/2(X2) -> [dq3]
  Tracking Differentiator 3/3(X3) -> [ddq3]
  Demux/3 -> Tracking Differentiator 3/1(Reference)
  Tracking Differentiator 4/1(X1) -> [q4]
  Tracking Differentiator 4/2(X2) -> [dq4]
  Tracking Differentiator 4/3(X3) -> [ddq4]
  Demux/4 -> Tracking Differentiator 4/1(Reference)
  Tracking Differentiator 5/1(X1) -> [q5]
  Tracking Differentiator 5/2(X2) -> [dq5]
  Tracking Differentiator 5/3(X3) -> [ddq5]
  Tracking Differentiator 6/1(X1) -> [q6]
  Tracking Differentiator 6/2(X2) -> [dq6]
  Tracking Differentiator 6/3(X3) -> [ddq6]
  Demux/5 -> Tracking Differentiator 5/1(Reference)
  Demux/6 -> Tracking Differentiator 6/1(Reference)
  Mux/1 -> qde/1
  [q1] -> Mux/1
  [q2] -> Mux/2
  [q4] -> Mux/4
  [q3] -> Mux/3
  [q6] -> Mux/6
  [q5] -> Mux/5
  Mux1/1 -> dqde/1
  [dq1] -> Mux1/1
  [dq2] -> Mux1/2
  [dq4] -> Mux1/4
  [dq3] -> Mux1/3
  [dq6] -> Mux1/6
  [dq5] -> Mux1/5
  Mux2/1 -> ddqde/1
  [ddq1] -> Mux2/1
  [ddq2] -> Mux2/2
  [ddq4] -> Mux2/4
  [ddq3] -> Mux2/3
  [ddq6] -> Mux2/6
  [ddq5] -> Mux2/5

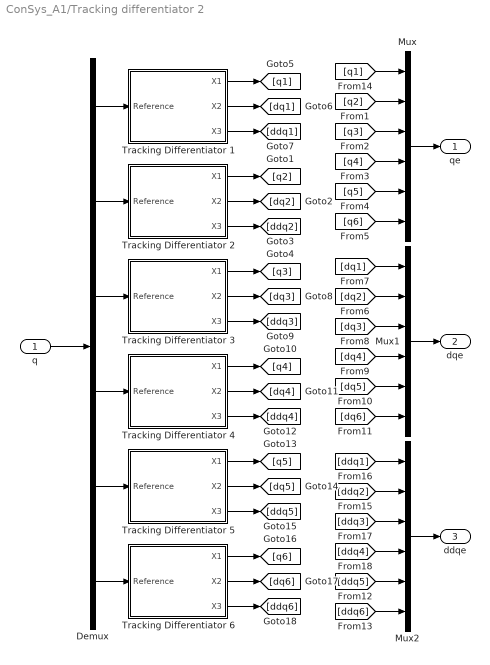
== system ConSys_A1/Tracking differentiator 2 ==
  q : Inport
  Demux : Demux  Outputs=6
  Mux : Mux  Inputs=6
  Mux1 : Mux  Inputs=6
  Mux2 : Mux  Inputs=6
  Tracking Differentiator 1 : Subsystem
  Tracking Differentiator 2 : Subsystem
  Tracking Differentiator 3 : Subsystem
  Tracking Differentiator 4 : Subsystem
  Tracking Differentiator 5 : Subsystem
  Tracking Differentiator 6 : Subsystem
  qe : Outport
  dqe : Outport  Port=2
  ddqe : Outport  Port=3
  wires:
  [ddq5] -> Mux2/5
  [ddq6] -> Mux2/6
  [ddq3] -> Mux2/3
  [ddq4] -> Mux2/4
  [ddq2] -> Mux2/2
  [ddq1] -> Mux2/1
  Mux2/1 -> ddqe/1
  [dq5] -> Mux1/5
  [dq6] -> Mux1/6
  [dq3] -> Mux1/3
  [dq4] -> Mux1/4
  [dq2] -> Mux1/2
  [dq1] -> Mux1/1
  Mux1/1 -> dqe/1
  [q5] -> Mux/5
  [q6] -> Mux/6
  [q3] -> Mux/3
  [q4] -> Mux/4
  [q2] -> Mux/2
  [q1] -> Mux/1
  Mux/1 -> qe/1
  Demux/6 -> Tracking Differentiator 6/1(Reference)
  Demux/5 -> Tracking Differentiator 5/1(Reference)
  Tracking Differentiator 6/3(X3) -> [ddq6]
  Tracking Differentiator 6/2(X2) -> [dq6]
  Tracking Differentiator 6/1(X1) -> [q6]
  Tracking Differentiator 5/3(X3) -> [ddq5]
  Tracking Differentiator 5/2(X2) -> [dq5]
  Tracking Differentiator 5/1(X1) -> [q5]
  Demux/4 -> Tracking Differentiator 4/1(Reference)
  Tracking Differentiator 4/3(X3) -> [ddq4]
  Tracking Differentiator 4/2(X2) -> [dq4]
  Tracking Differentiator 4/1(X1) -> [q4]
  Demux/3 -> Tracking Differentiator 3/1(Reference)
  Tracking Differentiator 3/3(X3) -> [ddq3]
  Tracking Differentiator 3/2(X2) -> [dq3]
  Tracking Differentiator 3/1(X1) -> [q3]
  Demux/2 -> Tracking Differentiator 2/1(Reference)
  Demux/1 -> Tracking Differentiator 1/1(Reference)
  q/1 -> Demux/1
  Tracking Differentiator 2/3(X3) -> [ddq2]
  Tracking Differentiator 2/2(X2) -> [dq2]
  Tracking Differentiator 2/1(X1) -> [q2]
  Tracking Differentiator 1/3(X3) -> [ddq1]
  Tracking Differentiator 1/2(X2) -> [dq1]
  Tracking Differentiator 1/1(X1) -> [q1]

== system ConSys_A1/Robot Arm ABB IRB-140/ADAMS Plant ==
  ADAMS inputs : Inport
  S-Function : S-Function  StopFcn=clear mex  FunctionName=adams_plant  Parameters=exevie,exesol,stat,outfil,nampre,o_rate,nam_in,namout,dft,modsim,modani,dt_out,inicmd,exetyp,comtyp,ada_host, workdir,pin_interp_order,pout_extrap_order,pin_extrap_order,pout_interp_order,simulink_lead_cosim  EnableBusSupport=off
  ADAMS outputs : Outport  InitialOutput=0
  wires:
  S-Function/1 -> ADAMS outputs/1
  ADAMS inputs/1 -> S-Function/1

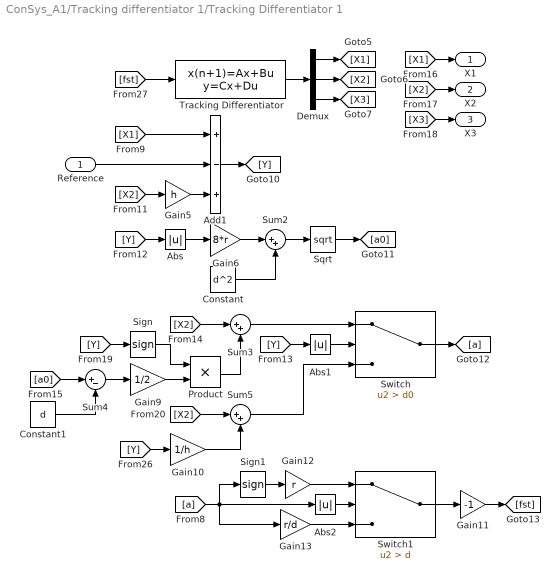
== system ConSys_A1/Tracking differentiator 1/Tracking Differentiator 1 ==
  Reference : Inport
  Abs : Abs
  Abs1 : Abs
  Abs2 : Abs
  Add1 : Sum  Inputs=+-+
  Constant : Constant  Value=d^2
  Constant1 : Constant  Value=d
  Demux : Demux  Outputs=3
  Gain10 : Gain  Gain=1/h
  Gain11 : Gain  Gain=-1
  Gain12 : Gain  Gain=r
  Gain13 : Gain  Gain=r/d
  Gain5 : Gain  Gain=h
  Gain6 : Gain  Gain=8*r
  Gain9 : Gain  Gain=1/2
  Product : Product
  Sign : Signum
  Sign1 : Signum
  Sqrt : Sqrt  SaturateOnIntegerOverflow=on
  Sum2 : Sum  Inputs=|++
  Sum3 : Sum  Inputs=|++
  Sum4 : Sum  Inputs=|+-
  Sum5 : Sum  Inputs=|++
  Switch : Switch  Criteria=u2 > Threshold  Threshold=d0
  Switch1 : Switch  Criteria=u2 > Threshold  Threshold=d
  Tracking Differentiator : DiscreteStateSpace  A=TD.a  B=TD.b  C=TD.c  D=TD.d  SampleTime=Ts
  X1 : Outport
  X2 : Outport  Port=2
  X3 : Outport  Port=3
  wires:
  [X3] -> X3/1
  Gain5/1 -> Add1/3
  [X1] -> Add1/1
  Gain12/1 -> Switch1/1
  [X2] -> X2/1
  [X2] -> Gain5/1
  Reference/1 -> Add1/2
  [X1] -> X1/1
  Add1/1 -> [Y]
  Demux/1 -> [X1]
  Demux/3 -> [X3]
  Tracking Differentiator/1 -> Demux/1
  Demux/2 -> [X2]
  [Y] -> Abs/1
  Gain6/1 -> Sum2/1
  Abs/1 -> Gain6/1
  Constant/1 -> Sum2/2
  Sqrt/1 -> [a0]
  Sum2/1 -> Sqrt/1
  Abs1/1 -> Switch/2
  Sign1/1 -> Gain12/1
  Gain9/1 -> Product/2
  [Y] -> Abs1/1
  Sum3/1 -> Switch/1
  [X2] -> Sum3/1
  Sum4/1 -> Gain9/1
  Gain13/1 -> Switch1/3
  [a0] -> Sum4/1
  Product/1 -> Sum3/2
  Sign/1 -> Product/1
  Constant1/1 -> Sum4/2
  [X2] -> Sum5/1
  [fst] -> Tracking Differentiator/1
  Gain10/1 -> Sum5/2
  [a] -> Gain13/1, Sign1/1, Abs2/1
  Switch1/1 -> Gain11/1
  [Y] -> Sign/1
  Switch/1 -> [a]
  Sum5/1 -> Switch/3
  [Y] -> Gain10/1
  Abs2/1 -> Switch1/2
  Gain11/1 -> [fst]

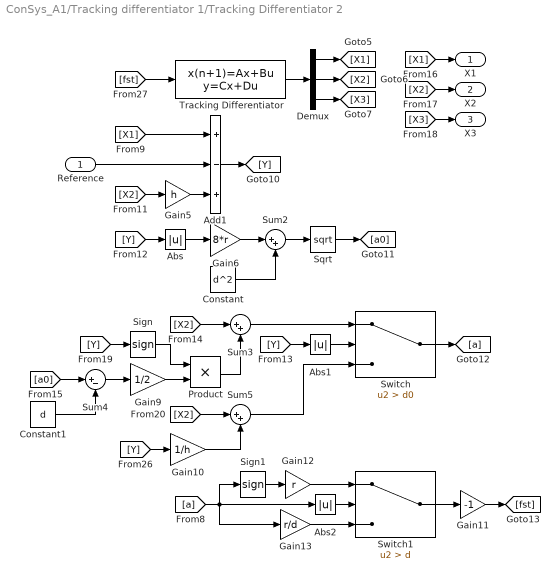
== system ConSys_A1/Tracking differentiator 1/Tracking Differentiator 2 ==
  Reference : Inport
  Abs : Abs
  Abs1 : Abs
  Abs2 : Abs
  Add1 : Sum  Inputs=+-+
  Constant : Constant  Value=d^2
  Constant1 : Constant  Value=d
  Demux : Demux  Outputs=3
  Gain10 : Gain  Gain=1/h
  Gain11 : Gain  Gain=-1
  Gain12 : Gain  Gain=r
  Gain13 : Gain  Gain=r/d
  Gain5 : Gain  Gain=h
  Gain6 : Gain  Gain=8*r
  Gain9 : Gain  Gain=1/2
  Product : Product
  Sign : Signum
  Sign1 : Signum
  Sqrt : Sqrt  SaturateOnIntegerOverflow=on
  Sum2 : Sum  Inputs=|++
  Sum3 : Sum  Inputs=|++
  Sum4 : Sum  Inputs=|+-
  Sum5 : Sum  Inputs=|++
  Switch : Switch  Criteria=u2 > Threshold  Threshold=d0
  Switch1 : Switch  Criteria=u2 > Threshold  Threshold=d
  Tracking Differentiator : DiscreteStateSpace  A=TD.a  B=TD.b  C=TD.c  D=TD.d  SampleTime=Ts
  X1 : Outport
  X2 : Outport  Port=2
  X3 : Outport  Port=3
  wires:
  Gain11/1 -> [fst]
  Abs2/1 -> Switch1/2
  [Y] -> Gain10/1
  Sum5/1 -> Switch/3
  Switch/1 -> [a]
  [Y] -> Sign/1
  Switch1/1 -> Gain11/1
  [a] -> Abs2/1, Sign1/1, Gain13/1
  Gain10/1 -> Sum5/2
  [fst] -> Tracking Differentiator/1
  [X2] -> Sum5/1
  Constant1/1 -> Sum4/2
  Sign/1 -> Product/1
  Product/1 -> Sum3/2
  [a0] -> Sum4/1
  Gain13/1 -> Switch1/3
  Sum4/1 -> Gain9/1
  [X2] -> Sum3/1
  Sum3/1 -> Switch/1
  [Y] -> Abs1/1
  Gain9/1 -> Product/2
  Sign1/1 -> Gain12/1
  Abs1/1 -> Switch/2
  Sum2/1 -> Sqrt/1
  Sqrt/1 -> [a0]
  Constant/1 -> Sum2/2
  Abs/1 -> Gain6/1
  Gain6/1 -> Sum2/1
  [Y] -> Abs/1
  Demux/2 -> [X2]
  Tracking Differentiator/1 -> Demux/1
  Demux/3 -> [X3]
  Demux/1 -> [X1]
  Add1/1 -> [Y]
  [X1] -> X1/1
  Reference/1 -> Add1/2
  [X2] -> Gain5/1
  [X2] -> X2/1
  Gain12/1 -> Switch1/1
  [X1] -> Add1/1
  Gain5/1 -> Add1/3
  [X3] -> X3/1

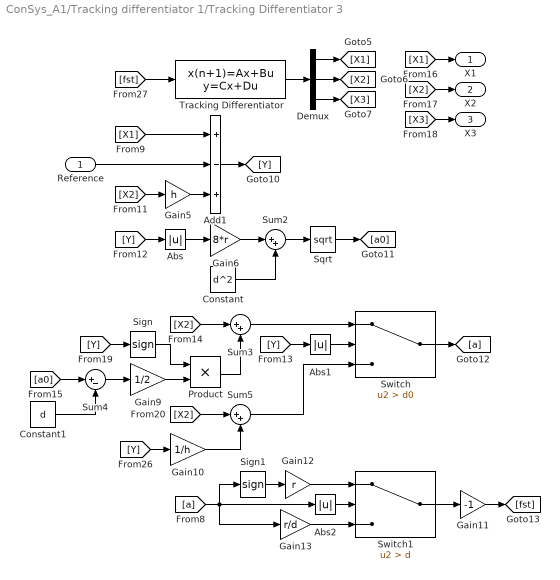
== system ConSys_A1/Tracking differentiator 1/Tracking Differentiator 3 ==
  Reference : Inport
  Abs : Abs
  Abs1 : Abs
  Abs2 : Abs
  Add1 : Sum  Inputs=+-+
  Constant : Constant  Value=d^2
  Constant1 : Constant  Value=d
  Demux : Demux  Outputs=3
  Gain10 : Gain  Gain=1/h
  Gain11 : Gain  Gain=-1
  Gain12 : Gain  Gain=r
  Gain13 : Gain  Gain=r/d
  Gain5 : Gain  Gain=h
  Gain6 : Gain  Gain=8*r
  Gain9 : Gain  Gain=1/2
  Product : Product
  Sign : Signum
  Sign1 : Signum
  Sqrt : Sqrt  SaturateOnIntegerOverflow=on
  Sum2 : Sum  Inputs=|++
  Sum3 : Sum  Inputs=|++
  Sum4 : Sum  Inputs=|+-
  Sum5 : Sum  Inputs=|++
  Switch : Switch  Criteria=u2 > Threshold  Threshold=d0
  Switch1 : Switch  Criteria=u2 > Threshold  Threshold=d
  Tracking Differentiator : DiscreteStateSpace  A=TD.a  B=TD.b  C=TD.c  D=TD.d  SampleTime=Ts
  X1 : Outport
  X2 : Outport  Port=2
  X3 : Outport  Port=3
  wires:
  [X3] -> X3/1
  Gain5/1 -> Add1/3
  [X1] -> Add1/1
  Gain12/1 -> Switch1/1
  [X2] -> X2/1
  [X2] -> Gain5/1
  Reference/1 -> Add1/2
  [X1] -> X1/1
  Add1/1 -> [Y]
  Demux/1 -> [X1]
  Demux/3 -> [X3]
  Tracking Differentiator/1 -> Demux/1
  Demux/2 -> [X2]
  [Y] -> Abs/1
  Gain6/1 -> Sum2/1
  Abs/1 -> Gain6/1
  Constant/1 -> Sum2/2
  Sqrt/1 -> [a0]
  Sum2/1 -> Sqrt/1
  Abs1/1 -> Switch/2
  Sign1/1 -> Gain12/1
  Gain9/1 -> Product/2
  [Y] -> Abs1/1
  Sum3/1 -> Switch/1
  [X2] -> Sum3/1
  Sum4/1 -> Gain9/1
  Gain13/1 -> Switch1/3
  [a0] -> Sum4/1
  Product/1 -> Sum3/2
  Sign/1 -> Product/1
  Constant1/1 -> Sum4/2
  [X2] -> Sum5/1
  [fst] -> Tracking Differentiator/1
  Gain10/1 -> Sum5/2
  [a] -> Gain13/1, Sign1/1, Abs2/1
  Switch1/1 -> Gain11/1
  [Y] -> Sign/1
  Switch/1 -> [a]
  Sum5/1 -> Switch/3
  [Y] -> Gain10/1
  Abs2/1 -> Switch1/2
  Gain11/1 -> [fst]

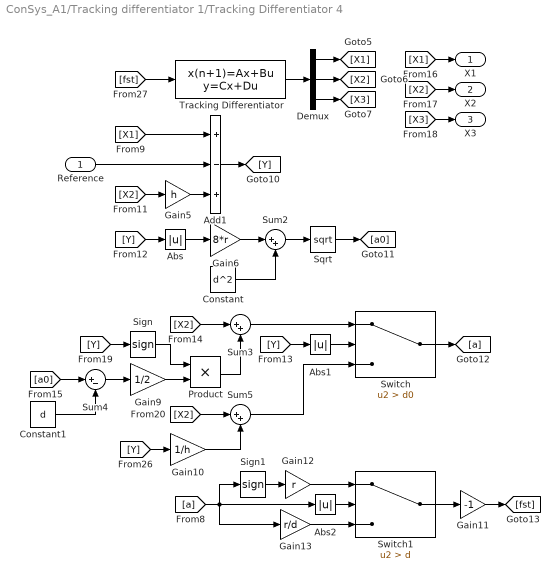
== system ConSys_A1/Tracking differentiator 1/Tracking Differentiator 4 ==
  Reference : Inport
  Abs : Abs
  Abs1 : Abs
  Abs2 : Abs
  Add1 : Sum  Inputs=+-+
  Constant : Constant  Value=d^2
  Constant1 : Constant  Value=d
  Demux : Demux  Outputs=3
  Gain10 : Gain  Gain=1/h
  Gain11 : Gain  Gain=-1
  Gain12 : Gain  Gain=r
  Gain13 : Gain  Gain=r/d
  Gain5 : Gain  Gain=h
  Gain6 : Gain  Gain=8*r
  Gain9 : Gain  Gain=1/2
  Product : Product
  Sign : Signum
  Sign1 : Signum
  Sqrt : Sqrt  SaturateOnIntegerOverflow=on
  Sum2 : Sum  Inputs=|++
  Sum3 : Sum  Inputs=|++
  Sum4 : Sum  Inputs=|+-
  Sum5 : Sum  Inputs=|++
  Switch : Switch  Criteria=u2 > Threshold  Threshold=d0
  Switch1 : Switch  Criteria=u2 > Threshold  Threshold=d
  Tracking Differentiator : DiscreteStateSpace  A=TD.a  B=TD.b  C=TD.c  D=TD.d  SampleTime=Ts
  X1 : Outport
  X2 : Outport  Port=2
  X3 : Outport  Port=3
  wires:
  Gain11/1 -> [fst]
  Abs2/1 -> Switch1/2
  [Y] -> Gain10/1
  Sum5/1 -> Switch/3
  Switch/1 -> [a]
  [Y] -> Sign/1
  Switch1/1 -> Gain11/1
  [a] -> Abs2/1, Sign1/1, Gain13/1
  Gain10/1 -> Sum5/2
  [fst] -> Tracking Differentiator/1
  [X2] -> Sum5/1
  Constant1/1 -> Sum4/2
  Sign/1 -> Product/1
  Product/1 -> Sum3/2
  [a0] -> Sum4/1
  Gain13/1 -> Switch1/3
  Sum4/1 -> Gain9/1
  [X2] -> Sum3/1
  Sum3/1 -> Switch/1
  [Y] -> Abs1/1
  Gain9/1 -> Product/2
  Sign1/1 -> Gain12/1
  Abs1/1 -> Switch/2
  Sum2/1 -> Sqrt/1
  Sqrt/1 -> [a0]
  Constant/1 -> Sum2/2
  Abs/1 -> Gain6/1
  Gain6/1 -> Sum2/1
  [Y] -> Abs/1
  Demux/2 -> [X2]
  Tracking Differentiator/1 -> Demux/1
  Demux/3 -> [X3]
  Demux/1 -> [X1]
  Add1/1 -> [Y]
  [X1] -> X1/1
  Reference/1 -> Add1/2
  [X2] -> Gain5/1
  [X2] -> X2/1
  Gain12/1 -> Switch1/1
  [X1] -> Add1/1
  Gain5/1 -> Add1/3
  [X3] -> X3/1

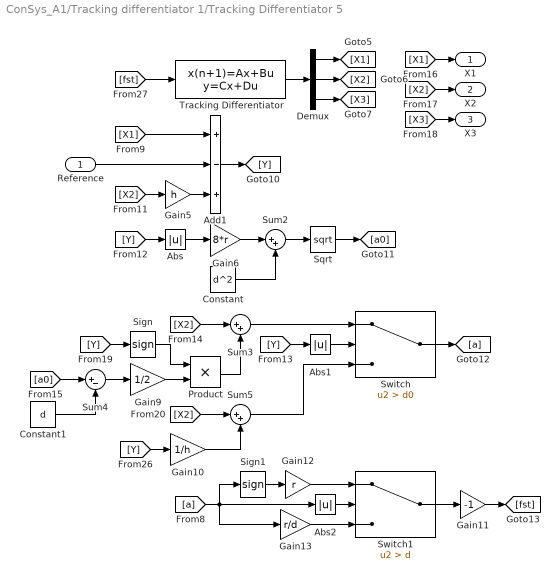
== system ConSys_A1/Tracking differentiator 1/Tracking Differentiator 5 ==
  Reference : Inport
  Abs : Abs
  Abs1 : Abs
  Abs2 : Abs
  Add1 : Sum  Inputs=+-+
  Constant : Constant  Value=d^2
  Constant1 : Constant  Value=d
  Demux : Demux  Outputs=3
  Gain10 : Gain  Gain=1/h
  Gain11 : Gain  Gain=-1
  Gain12 : Gain  Gain=r
  Gain13 : Gain  Gain=r/d
  Gain5 : Gain  Gain=h
  Gain6 : Gain  Gain=8*r
  Gain9 : Gain  Gain=1/2
  Product : Product
  Sign : Signum
  Sign1 : Signum
  Sqrt : Sqrt  SaturateOnIntegerOverflow=on
  Sum2 : Sum  Inputs=|++
  Sum3 : Sum  Inputs=|++
  Sum4 : Sum  Inputs=|+-
  Sum5 : Sum  Inputs=|++
  Switch : Switch  Criteria=u2 > Threshold  Threshold=d0
  Switch1 : Switch  Criteria=u2 > Threshold  Threshold=d
  Tracking Differentiator : DiscreteStateSpace  A=TD.a  B=TD.b  C=TD.c  D=TD.d  SampleTime=Ts
  X1 : Outport
  X2 : Outport  Port=2
  X3 : Outport  Port=3
  wires:
  [X3] -> X3/1
  Gain5/1 -> Add1/3
  [X1] -> Add1/1
  Gain12/1 -> Switch1/1
  [X2] -> X2/1
  [X2] -> Gain5/1
  Reference/1 -> Add1/2
  [X1] -> X1/1
  Add1/1 -> [Y]
  Demux/1 -> [X1]
  Demux/3 -> [X3]
  Tracking Differentiator/1 -> Demux/1
  Demux/2 -> [X2]
  [Y] -> Abs/1
  Gain6/1 -> Sum2/1
  Abs/1 -> Gain6/1
  Constant/1 -> Sum2/2
  Sqrt/1 -> [a0]
  Sum2/1 -> Sqrt/1
  Abs1/1 -> Switch/2
  Sign1/1 -> Gain12/1
  Gain9/1 -> Product/2
  [Y] -> Abs1/1
  Sum3/1 -> Switch/1
  [X2] -> Sum3/1
  Sum4/1 -> Gain9/1
  Gain13/1 -> Switch1/3
  [a0] -> Sum4/1
  Product/1 -> Sum3/2
  Sign/1 -> Product/1
  Constant1/1 -> Sum4/2
  [X2] -> Sum5/1
  [fst] -> Tracking Differentiator/1
  Gain10/1 -> Sum5/2
  [a] -> Gain13/1, Sign1/1, Abs2/1
  Switch1/1 -> Gain11/1
  [Y] -> Sign/1
  Switch/1 -> [a]
  Sum5/1 -> Switch/3
  [Y] -> Gain10/1
  Abs2/1 -> Switch1/2
  Gain11/1 -> [fst]
